simulink model "first_model_simulink"  (R2023a)
settings: Solver=VariableStepAuto  StartTime=0.0  StopTime=sim_time  MaxStep=1  RelTol=1e-3
values from neighbouring files (symbols this model uses):
  A_f = 2    [parameter_definiciton.m]
  air_dens = 1.22521    [parameter_definiciton.m]
  angle_road = atan(slope_road/100)    [parameter_definiciton.m]
  C_d = 0.35    [parameter_definiciton.m]
  f_r = 0.017    [parameter_definiciton.m]
  g = 9.8    [parameter_definiciton.m]
  m_v = 1000    [parameter_definiciton.m]
  wind_speed = 0    [parameter_definiciton.m]
libraries: simulink x1
settings Model: Creator=citcea  LastModifiedBy=citcea

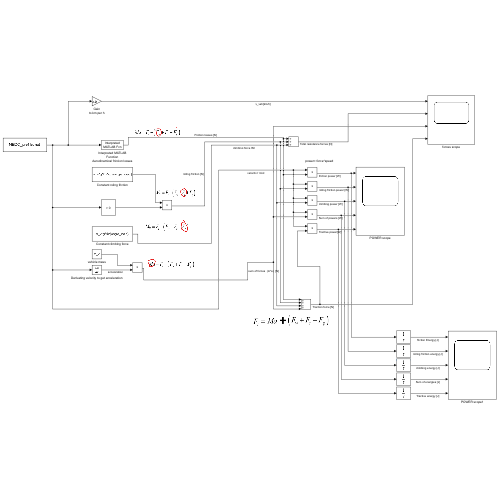
[thumbnail: Simulink's stored preview of the top-level diagram]
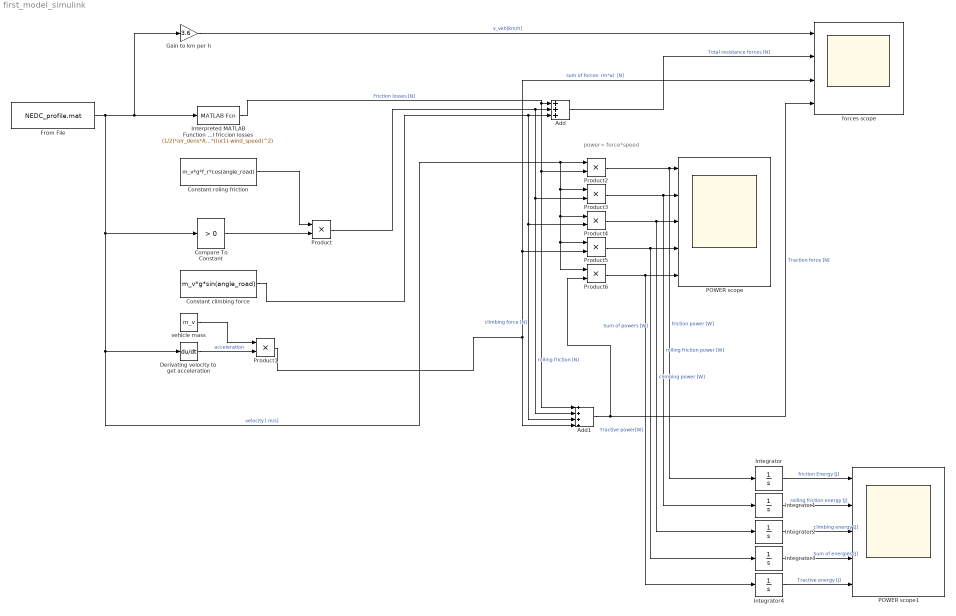
== system first_model_simulink ==
  note: power= force*speed
  Add : Sum  Inputs=+++
  Add1 : Sum  Inputs=++++
  Compare To Constant : simulink/Logic and Bit Operations/Compare To Constant  relop=>  const=0  OutDataTypeStr=boolean
  Constant climbing force : Constant  Value=m_v*g*sin(angle_road)
  Constant roling friction : Constant  Value=m_v*g*f_r*cos(angle_road)
  Derivating velocity to get acceleration : Derivative
  From File : FromFile  FileName=NEDC_profile.mat  SampleTime=0
  Gain to km per h : Gain  Gain=3.6
  Integrator{,1..4} (5 alike) : Integrator
  Interpreted MATLAB Function Aerodinamical friccion losses : MATLABFcn  MATLABFcn=(1/2)*air_dens*A_f*C_d*((u(1)-wind_speed)^2)
  POWER scope : Scope  NumInputPorts=5
  POWER scope1 : Scope  NumInputPorts=5
  Product{,1..6} (7 alike) : Product
  forces scope : Scope  NumInputPorts=4
  vehicle mass : Constant  Value=m_v
  wires:
  Interpreted MATLAB Function Aerodinamical friccion losses/1 -> Product2/2, Add1/1, Add/1  "Friction losses [N]"
  Gain to km per h/1 -> forces scope/1  "v_veh[km/h]"
  Compare To Constant/1 -> Product/2
  Constant roling friction/1 -> Product/1
  Product/1 -> Product3/2, Add1/2, Add/2  "rolling friction [N]"
  Constant climbing force/1 -> Product4/2, Add1/3, Add/3  "climbing force [N]"
  Add/1 -> forces scope/2  "Total resistance forces [N]"
  vehicle mass/1 -> Product1/1
  Derivating velocity to get acceleration/1 -> Product1/2  "acceleration"
  Product1/1 -> Product5/2, forces scope/3, Add1/4  "sum of forces  (m*a)  [N]"
  Add1/1 -> Product6/2, forces scope/4  "Traction force [N]"
  From File/1 -> Derivating velocity to get acceleration/1, Product6/1, Product5/1, Product4/1, Product3/1, Product2/1, Compare To Constant/1, Gain to km per h/1, Interpreted MATLAB Function Aerodinamical friccion losses/1  "velocity [ m/s]"
  Product2/1 -> Integrator/1, POWER scope/1  "friction power [W]"
  Product4/1 -> Integrator2/1, POWER scope/3  "climbing power [W]"
  Product5/1 -> Integrator3/1, POWER scope/4  "Sum of powers [W]"
  Product3/1 -> Integrator1/1, POWER scope/2  "rolling friction power [W]"
  Product6/1 -> Integrator4/1, POWER scope/5  "Tractive power[W]"
  Integrator/1 -> POWER scope1/1  "friction Energy [J]"
  Integrator1/1 -> POWER scope1/2  "rolling friction energy [J]"
  Integrator2/1 -> POWER scope1/3  "climbing energy [J]"
  Integrator3/1 -> POWER scope1/4  "Sum of energies [J]"
  Integrator4/1 -> POWER scope1/5  "Tractive energy [J]"
